simulink model "tank1_closed_loop"  (R2026a)
settings: Solver=VariableStepAuto  StopTime=7
libraries: slpidlib x1

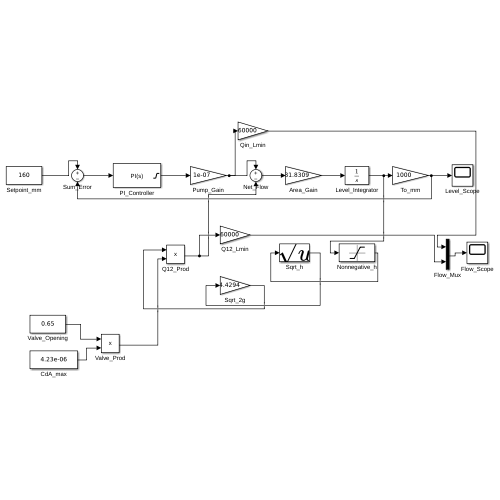
[thumbnail: Simulink's stored preview of the top-level diagram]
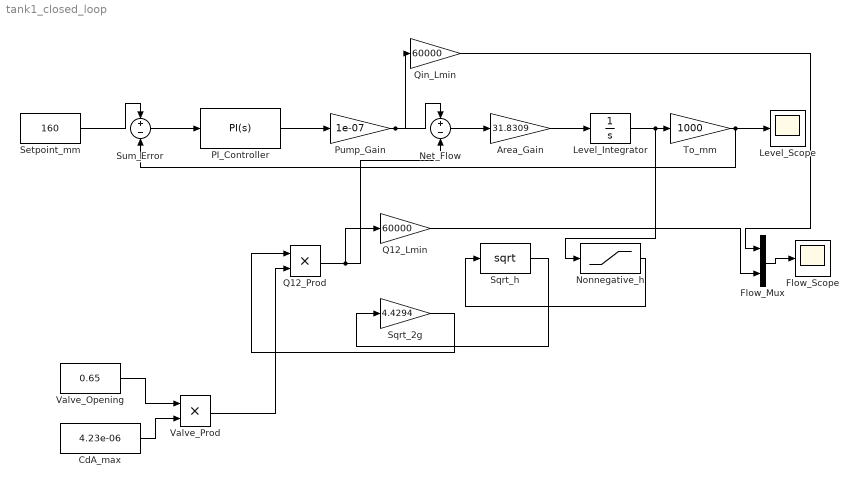
== system tank1_closed_loop ==
  Area_Gain : Gain  Gain=31.8309
  CdA_max : Constant  Value=4.23e-06
  Flow_Mux : Mux  Inputs=2
  Flow_Scope : Scope
  Level_Integrator : Integrator  InitialCondition=0.16
  Level_Scope : Scope
  Net_Flow : Sum  Inputs=+-
  Nonnegative_h : Saturate  UpperLimit=inf  LowerLimit=0
  PI_Controller : slpidlib/PID Controller  Controller=PI  Form=Parallel  TimeDomain=Continuous-time  UseExternalTs=off  SampleTime=-1  IntegratorMethod=Forward Euler  FilterMethod=Forward Euler  ControllerParametersSource=internal  P=1.2  I=0.008  UseKiTs=off  D=0  UseExternalDerivativeSource=off  N=100  UseFilter=on  TunerSelectOption=Transfer Function Based (PID Tuner App)  InitialConditionSource=internal  InitialConditionForIntegrator=0  InitialConditionForFilter=0  DifferentiatorICPrevScaledInput=0  ExternalReset=none  TrackingMode=off  Kt=1  LimitOutput=on  SatLimitsSource=internal  UpperSaturationLimit=100  LowerSaturationLimit=0  LinearizeAsGain=on  AntiWindupMode=none  Kb=1  LimitIntegrator=off  UpperIntegratorSaturationLimit=inf  LowerIntegratorSaturationLimit=-inf  POutMin=[]  POutMax=[]  IOutMin=[]  IOutMax=[]  DOutMin=[]  DOutMax=[]  NOutMin=[]  NOutMax=[]  SumOutMin=[]  SumOutMax=[]  SaturationOutMin=[]  SaturationOutMax=[]  PParamMin=[]  PParamMax=[]  IParamMin=[]  IParamMax=[]  DParamMin=[]  DParamMax=[]  NParamMin=[]  NParamMax=[]  KbParamMin=[]  KbParamMax=[]  KtParamMin=[]  KtParamMax=[]  KbOutMin=[]  KbOutMax=[]  KtOutMin=[]  KtOutMax=[]  IntegratorOutMin=[]  IntegratorOutMax=[]  FilterOutMin=[]  FilterOutMax=[]  SumI1OutMin=[]  SumI1OutMax=[]  SumI2OutMin=[]  SumI2OutMax=[]  SumI3OutMin=[]  SumI3OutMax=[]  SumI4OutMin=[]  SumI4OutMax=[]  SumDOutMin=[]  SumDOutMax=[]  DifferentiatorOutMin=[]  DifferentiatorOutMax=[]  FilterDiffOutCoefMin=[]  FilterDiffOutCoefMax=[]  ReciprocalOutMin=[]  ReciprocalOutMax=[]  SumDenOutMin=[]  SumDenOutMax=[]  SumNumOutMin=[]  SumNumOutMax=[]  DivideOutMin=[]  DivideOutMax=[]  UdiffTsProdOutMin=[]  UdiffTsProdOutMax=[]  NTsProdOutMin=[]  NTsProdOutMax=[]  UintegralTsProdOutMin=[]  UintegralTsProdOutMax=[]  UngainTsProdOutMin=[]  UngainTsProdOutMax=[]  ClampingZeroOutDataTypeStr=Inherit: Inherit via back propagation  ClampingZeroOutMin=[]  ClampingZeroOutMax=[]  FilterDenConstantOutDataTypeStr=Inherit: Inherit via back propagation  FilterDenConstantOutMin=[]  FilterDenConstantOutMax=[]  PCopyOutDataTypeStr=Inherit: Inherit via back propagation  PCopyOutMin=[]  PCopyOutMax=[]  NCopyOutDataTypeStr=Inherit: Inherit via back propagation  NCopyOutMin=[]  NCopyOutMax=[]  IntegratorContinuousStateAttributes=''  IntegratorStateMustResolveToSignalObject=off  IntegratorRTWStateStorageClass=Auto  FilterContinuousStateAttributes=''  FilterStateMustResolveToSignalObject=off  FilterRTWStateStorageClass=Auto  ParallelPVariant=InternalParameters  IdealPVariant=Disabled  IVariant=InternalParameters  DVariant=Disabled  IntegratorVariant=Continuous  SatVariant=Enabled  AWVariant=Passthrough  PCopyVariant=Disabled  TRVariant=Disabled  FdbkBlocksVariant=Forward  IdealPFdbkVariant=Disabled  SatFdbkVariant=Disabled  DerivativeFilterVariant=Disabled  NVariant=Disabled  NCopyVariant=Disabled_SignalSpec  FilterICVariant=Disabled  IntegratorICVariant=InternalICs  ExternalResetVariant=Disabled  TRSumVariant=Passthrough  SumFdbkVariant=Disabled  SumVariant=Sum_PI  TsampFilterVariant=InternalTs  TsampNgainVariant=Passthrough  TsampIntegralVariant=Disabled_SignalSpec  ExternalSaturationOutDataTypeStr=Inherit: Same as second input  DerivativeSourceVariant=Disabled  PreIntVariant=InternalPreInt
  Pump_Gain : Gain  Gain=1e-07
  Q12_Lmin : Gain  Gain=60000
  Q12_Prod : Product
  Qin_Lmin : Gain  Gain=60000
  Setpoint_mm : Constant  Value=160
  Sqrt_2g : Gain  Gain=4.4294
  Sqrt_h : Math  Operator=sqrt
  Sum_Error : Sum  Inputs=+-
  To_mm : Gain  Gain=1000
  Valve_Opening : Constant  Value=0.65
  Valve_Prod : Product
  wires:
  Setpoint_mm/1 -> Sum_Error/1
  Sum_Error/1 -> PI_Controller/1
  PI_Controller/1 -> Pump_Gain/1
  Pump_Gain/1 -> Net_Flow/1, Qin_Lmin/1
  Net_Flow/1 -> Area_Gain/1
  Area_Gain/1 -> Level_Integrator/1
  Level_Integrator/1 -> To_mm/1, Nonnegative_h/1
  To_mm/1 -> Level_Scope/1, Sum_Error/2
  Nonnegative_h/1 -> Sqrt_h/1
  Sqrt_h/1 -> Sqrt_2g/1
  Sqrt_2g/1 -> Q12_Prod/1
  Valve_Opening/1 -> Valve_Prod/1
  CdA_max/1 -> Valve_Prod/2
  Valve_Prod/1 -> Q12_Prod/2
  Q12_Prod/1 -> Net_Flow/2, Q12_Lmin/1
  Qin_Lmin/1 -> Flow_Mux/1
  Q12_Lmin/1 -> Flow_Mux/2
  Flow_Mux/1 -> Flow_Scope/1
